simulink model "bldc_sim_combined_2024"  (R2025a)
settings: Solver=VariableStepAuto  StartTime=0.0  StopTime=1.5  RelTol=1e-3
values from neighbouring files (symbols this model uses):
  phi_corr_LUT_param = Simulink.Parameter(phi_corr_LUT)    [lut_script.m]
undefined symbols (not defined in the file or in its folder): closed_loop, D_duty_cycle, D_m, DiscIntNeverNeededParam, hall_errors, I_duty_cycle, J_t, L_ss, lambda_m, P, P_duty_cycle, r_s, R_vs, T_m, theta_v, use_LUT, V_bus
libraries: spsMosfetLib x6, spsSeriesRLCBranchLib x4, spsVoltageMeasurementLib x3, spsControlledCurrentSourceLib x3, slpidlib x2, eeGeneralControl x1, simulink x1, embmathops x1, spsControlledVoltageSourceLib x1, spsPWMGeneratorDCDCLib x1, spsDCVoltageSourceLib x1, sps_lib x1
(part 1 of 2)
settings Model: Creator=Aether  LastModifiedBy=rnashota.stu

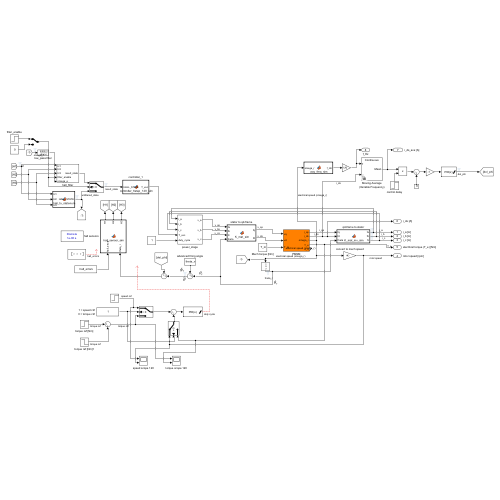
[thumbnail: Simulink's stored preview of the top-level diagram]
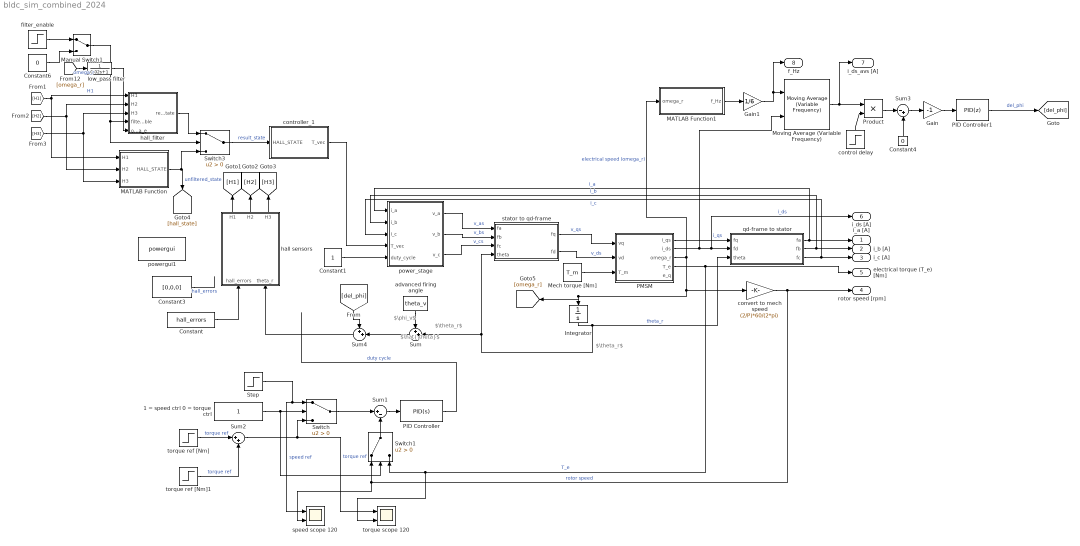
== system bldc_sim_combined_2024 ==
  note: $\theta_r$
  note: $\hat{\theta}$
  note: $\theta_r$
  note: $\phi_v$
  1 = speed ctrl 0 = torque ctrl : Constant
  Constant : Constant  Value=hall_errors
  Constant1 : Constant
  Constant3 : Constant  Value=[0,0,0]
  Constant4 : Constant  Value=0
  Constant6 : Constant  Value=0
  Gain : Gain  Gain=-1
  Gain1 : Gain  Gain=1/6
  Integrator : Integrator
  MATLAB Function : MATLAB Function  TreatAsAtomicUnit=on
  MATLAB Function1 : MATLAB Function  TreatAsAtomicUnit=on
  Manual Switch1 : ManualSwitch
  Mech torque [Nm] : Constant  Value=T_m
  Moving Average (Variable Frequency) : eeGeneralControl/Moving Average (Variable Frequency)  VariantControl=Variant1  LabelModeActiveChoice=Continuous  f0=60  fmin=1  x0=0  BufferSize=32768  Ts=0
      settings: LibrarySourceBlock=|
      | ee_sl_lib/General Control/Moving Average
      | (Variable Frequency)
  PID Controller : slpidlib/PID Controller  Controller=PID  Form=Parallel  TimeDomain=Continuous-time  UseExternalTs=off  SampleTime=-1  IntegratorMethod=Forward Euler  FilterMethod=Forward Euler  ControllerParametersSource=internal  P=P_duty_cycle  I=I_duty_cycle  UseKiTs=off  D=D_duty_cycle  UseExternalDerivativeSource=off  N=100  UseFilter=on  TunerSelectOption=Transfer Function Based (PID Tuner App)  InitialConditionSource=internal  InitialConditionForIntegrator=0  InitialConditionForFilter=0  DifferentiatorICPrevScaledInput=0  ExternalReset=none  TrackingMode=off  Kt=1  LimitOutput=on  SatLimitsSource=internal  UpperSaturationLimit=1  LowerSaturationLimit=0  LinearizeAsGain=on  AntiWindupMode=none  Kb=1  LimitIntegrator=off  UpperIntegratorSaturationLimit=inf  LowerIntegratorSaturationLimit=-inf  POutMin=[]  POutMax=[]  IOutMin=[]  IOutMax=[]  DOutMin=[]  DOutMax=[]  NOutMin=[]  NOutMax=[]  SumOutMin=[]  SumOutMax=[]  SaturationOutMin=[]  SaturationOutMax=[]  PParamMin=[]  PParamMax=[]  IParamMin=[]  IParamMax=[]  DParamMin=[]  DParamMax=[]  NParamMin=[]  NParamMax=[]  KbParamMin=[]  KbParamMax=[]  KtParamMin=[]  KtParamMax=[]  KbOutMin=[]  KbOutMax=[]  KtOutMin=[]  KtOutMax=[]  IntegratorOutMin=[]  IntegratorOutMax=[]  FilterOutMin=[]  FilterOutMax=[]  SumI1OutMin=[]  SumI1OutMax=[]  SumI2OutMin=[]  SumI2OutMax=[]  SumI3OutMin=[]  SumI3OutMax=[]  SumI4OutMin=[]  SumI4OutMax=[]  SumDOutMin=[]  SumDOutMax=[]  DifferentiatorOutMin=[]  DifferentiatorOutMax=[]  FilterDiffOutCoefMin=[]  FilterDiffOutCoefMax=[]  ReciprocalOutMin=[]  ReciprocalOutMax=[]  SumDenOutMin=[]  SumDenOutMax=[]  SumNumOutMin=[]  SumNumOutMax=[]  DivideOutMin=[]  DivideOutMax=[]  UdiffTsProdOutMin=[]  UdiffTsProdOutMax=[]  NTsProdOutMin=[]  NTsProdOutMax=[]  UintegralTsProdOutMin=[]  UintegralTsProdOutMax=[]  UngainTsProdOutMin=[]  UngainTsProdOutMax=[]  ClampingZeroOutDataTypeStr=Inherit: Inherit via back propagation  ClampingZeroOutMin=[]  ClampingZeroOutMax=[]  FilterDenConstantOutDataTypeStr=Inherit: Inherit via back propagation  FilterDenConstantOutMin=[]  FilterDenConstantOutMax=[]  PCopyOutDataTypeStr=Inherit: Inherit via back propagation  PCopyOutMin=[]  PCopyOutMax=[]  NCopyOutDataTypeStr=Inherit: Inherit via back propagation  NCopyOutMin=[]  NCopyOutMax=[]  IntegratorContinuousStateAttributes=''  IntegratorStateMustResolveToSignalObject=off  IntegratorRTWStateStorageClass=Auto  FilterContinuousStateAttributes=''  FilterStateMustResolveToSignalObject=off  FilterRTWStateStorageClass=Auto  ParallelPVariant=InternalParameters  IdealPVariant=Disabled  IVariant=InternalParameters  DVariant=InternalParameters  IntegratorVariant=Continuous  SatVariant=Enabled  AWVariant=Passthrough  PCopyVariant=Disabled  TRVariant=Disabled  FdbkBlocksVariant=Forward  IdealPFdbkVariant=Disabled  SatFdbkVariant=Disabled  DerivativeFilterVariant=ContFilter  NVariant=InternalParameters  NCopyVariant=Disabled  FilterICVariant=InternalICsFilter  IntegratorICVariant=InternalICs  ExternalResetVariant=Disabled  TRSumVariant=Passthrough  SumFdbkVariant=Disabled  SumVariant=Sum_PID  TsampFilterVariant=InternalTs  TsampNgainVariant=Passthrough  TsampIntegralVariant=Disabled_SignalSpec  ExternalSaturationOutDataTypeStr=Inherit: Same as second input  DerivativeSourceVariant=ErrorSignal  PreIntVariant=InternalPreInt
  PID Controller1 : slpidlib/PID Controller  Controller=PID  Form=Parallel  TimeDomain=Discrete-time  UseExternalTs=off  SampleTime=-1  IntegratorMethod=Forward Euler  FilterMethod=Forward Euler  ControllerParametersSource=internal  P=0.0068  I=0.744  UseKiTs=off  D=0  UseExternalDerivativeSource=off  N=100  UseFilter=on  TunerSelectOption=Transfer Function Based (PID Tuner App)  InitialConditionSource=internal  InitialConditionForIntegrator=0  InitialConditionForFilter=0  DifferentiatorICPrevScaledInput=0  ExternalReset=none  TrackingMode=off  Kt=1  LimitOutput=on  SatLimitsSource=internal  UpperSaturationLimit=pi/3  LowerSaturationLimit=-pi/3  LinearizeAsGain=on  AntiWindupMode=none  Kb=1  LimitIntegrator=off  UpperIntegratorSaturationLimit=inf  LowerIntegratorSaturationLimit=-inf  POutMin=[]  POutMax=[]  IOutMin=[]  IOutMax=[]  DOutMin=[]  DOutMax=[]  NOutMin=[]  NOutMax=[]  SumOutMin=[]  SumOutMax=[]  SaturationOutMin=[]  SaturationOutMax=[]  PParamMin=[]  PParamMax=[]  IParamMin=[]  IParamMax=[]  DParamMin=[]  DParamMax=[]  NParamMin=[]  NParamMax=[]  KbParamMin=[]  KbParamMax=[]  KtParamMin=[]  KtParamMax=[]  KbOutMin=[]  KbOutMax=[]  KtOutMin=[]  KtOutMax=[]  IntegratorOutMin=[]  IntegratorOutMax=[]  FilterOutMin=[]  FilterOutMax=[]  SumI1OutMin=[]  SumI1OutMax=[]  SumI2OutMin=[]  SumI2OutMax=[]  SumI3OutMin=[]  SumI3OutMax=[]  SumI4OutMin=[]  SumI4OutMax=[]  SumDOutMin=[]  SumDOutMax=[]  DifferentiatorOutMin=[]  DifferentiatorOutMax=[]  FilterDiffOutCoefMin=[]  FilterDiffOutCoefMax=[]  ReciprocalOutMin=[]  ReciprocalOutMax=[]  SumDenOutMin=[]  SumDenOutMax=[]  SumNumOutMin=[]  SumNumOutMax=[]  DivideOutMin=[]  DivideOutMax=[]  UdiffTsProdOutMin=[]  UdiffTsProdOutMax=[]  NTsProdOutMin=[]  NTsProdOutMax=[]  UintegralTsProdOutMin=[]  UintegralTsProdOutMax=[]  UngainTsProdOutMin=[]  UngainTsProdOutMax=[]  ClampingZeroOutDataTypeStr=Inherit: Inherit via back propagation  ClampingZeroOutMin=[]  ClampingZeroOutMax=[]  FilterDenConstantOutDataTypeStr=Inherit: Inherit via back propagation  FilterDenConstantOutMin=[]  FilterDenConstantOutMax=[]  PCopyOutDataTypeStr=Inherit: Inherit via back propagation  PCopyOutMin=[]  PCopyOutMax=[]  NCopyOutDataTypeStr=Inherit: Inherit via back propagation  NCopyOutMin=[]  NCopyOutMax=[]  IntegratorContinuousStateAttributes=''  IntegratorStateMustResolveToSignalObject=off  IntegratorRTWStateStorageClass=Auto  FilterContinuousStateAttributes=''  FilterStateMustResolveToSignalObject=off  FilterRTWStateStorageClass=Auto  ParallelPVariant=InternalParameters  IdealPVariant=Disabled  IVariant=InternalParameters  DVariant=InternalParameters  IntegratorVariant=Discrete  SatVariant=Enabled  AWVariant=Passthrough  PCopyVariant=Disabled  TRVariant=Disabled  FdbkBlocksVariant=Forward  IdealPFdbkVariant=Disabled  SatFdbkVariant=Disabled  DerivativeFilterVariant=ForwardEulerFilter  NVariant=InternalParameters  NCopyVariant=Disabled  FilterICVariant=InternalICsFilter  IntegratorICVariant=InternalICs  ExternalResetVariant=Disabled  TRSumVariant=Passthrough  SumFdbkVariant=Disabled  SumVariant=Sum_PID  TsampFilterVariant=InternalTs  TsampNgainVariant=Passthrough  TsampIntegralVariant=Disabled_SignalSpec  ExternalSaturationOutDataTypeStr=Inherit: Same as second input  DerivativeSourceVariant=ErrorSignal  PreIntVariant=InternalPreInt
  PMSM : Subsystem
  Product : Product
  Step : Step  Time=0.1  After=1000  SampleTime=0
  Sum : Sum  Inputs=++|
  Sum1 : Sum  Inputs=|+-
  Sum2 : Sum  Inputs=|++
  Sum3 : Sum  Inputs=|-+
  Sum4 : Sum  Inputs=++|
  Switch : Switch  Criteria=u2 > Threshold  SaturateOnIntegerOverflow=off  InputSameDT=off
  Switch1 : Switch  Criteria=u2 > Threshold  SaturateOnIntegerOverflow=off  InputSameDT=off
  Switch3 : Switch  Criteria=u2 > Threshold  SaturateOnIntegerOverflow=off  InputSameDT=off
  advanced firing angle : Constant  Value=theta_v
  control delay : Step  Time=0.6  SampleTime=0
  controller_1 : MATLAB Function  TreatAsAtomicUnit=on
  convert to mech speed : Gain  Gain=(2/P)*60/(2*pi)
  filter_enable : Step  Time=0.5  SampleTime=0
  hall sensors : MATLAB Function  TreatAsAtomicUnit=on
  hall_filter : Subsystem
  low_pass filter : TransferFcn  Denominator=[0.02 1]
  power_stage : Subsystem
  powergui1 : sps_lib/powergui  Priority=1  SimulationMode=Discrete  SampleTime=1e-6  frequency=60  Iterations=50  frequencyindice=0  Pbase=100e6  ErrMax=1e-4  UnitsV=kV  UnitsW=MW  buscounter=0  FunctionMessages=off  echomessages=off  EnableUseOfTLC=off  CurrentSourceSwitches=off  DisableSnubberDevices=off  DisableRonSwitches=off  DisableVfSwitches=off  DisplayEquations=off  AutomaticDiscreteSolvers=off  SolverType=Tustin/Backward Euler (TBE)  Interpol=off  ExternalGateDelay=off  methode=off  Ts=100  x0status=blocks  SPID=on  SwTol=0  HookPort=off  NonlinearTolerance=1e-4  nMaxIteration=100  ContinueOnMaxIteration=off  RestoreLinks=warning  ResistiveCurrentMeasurement=off  Frange=[0:2:500]  Ylog=off  Xlog=on  ShowGrid=off  save=off  variable=ZData  structure=0  ZoomFFT=off  StartTime=0.0  cycles=1  DisplayStyle=1  fundamental=60  FreqAxis=off  MaxFrequency=1000  frequencyindicesteady=1  RmsSteady=1  display=off
  qd-frame to stator : MATLAB Function  TreatAsAtomicUnit=on
  speed scope 120 : Scope  NumInputPorts=2
      settings: ActiveDisplayYMinimum=-1.1385486491945782E+15  ActiveDisplayYMaximum=1.0246937842751196E+16
  stator to qd-frame : MATLAB Function  TreatAsAtomicUnit=on
  torque ref [Nm] : Step  Time=0.1  After=1e-1  SampleTime=0  ZeroCross=off
  torque ref [Nm]1 : Step  After=-0.5e-1  SampleTime=0
  torque scope 120 : Scope  NumInputPorts=2
      settings: ActiveDisplayYMinimum=-0.89883  ActiveDisplayYMaximum=8.08945
  i_a [A] : Outport
  i_b [A] : Outport  Port=2
  i_c [A] : Outport  Port=3
  rotor speed [rpm] : Outport  Port=4
  electrical torque (T_e) [Nm] : Outport  Port=5
  i_ds [A] : Outport  Port=6
  i_ds_avs [A] : Outport  Port=7
  f_Hz : Outport  Port=8
  wires:
  Constant3/1 -> ?  "hall_errors"
  qd-frame to stator/2(fb) -> power_stage/2(i_b), i_b [A]/1  "i_b"
  qd-frame to stator/3(fc) -> power_stage/3(i_c), i_c [A]/1  "i_c"
  power_stage/1(v_a) -> stator to qd-frame/1(fa)  "v_as"
  Sum/1 -> Sum4/2
  PMSM/3(omega_r) -> MATLAB Function1/1(omega_r), convert to mech speed/1, [omega_r], Integrator/1  "electrical speed (omega_r)"
  Sum4/1 -> hall sensors/2(theta_r)
  advanced firing angle/1 -> Sum/1
  qd-frame to stator/1(fa) -> power_stage/1(i_a), i_a [A]/1  "i_a"
  Integrator/1 -> stator to qd-frame/4(theta), Sum/2, qd-frame to stator/3(theta)  "theta_r"
  power_stage/2(v_b) -> stator to qd-frame/2(fb)  "v_bs"
  stator to qd-frame/2(fd) -> PMSM/2(vd)  "v_ds"
  power_stage/3(v_c) -> stator to qd-frame/3(fc)  "v_cs"
  Mech torque [Nm]/1 -> PMSM/3(T_m)
  stator to qd-frame/1(fq) -> PMSM/1(vq)  "v_qs"
  PMSM/1(i_qs) -> qd-frame to stator/1(fq)  "i_qs"
  Product/1 -> Sum3/1
  Gain/1 -> PID Controller1/1
  Sum3/1 -> Gain/1
  PID Controller1/1 -> [del_phi]  "del_phi"
  Moving Average (Variable Frequency)/1 -> Product/1, i_ds_avs [A]/1
  PMSM/2(i_ds) -> qd-frame to stator/2(fd), i_ds [A]/1, Moving Average (Variable Frequency)/2  "i_ds"
  Constant4/1 -> Sum3/2
  control delay/1 -> Product/2
  [del_phi] -> Sum4/1
  Step/1 -> speed scope 120/1, Switch/1  "speed ref"
  1 = speed ctrl 0 = torque ctrl/1 -> Switch/2, Switch1/2
  Switch/1 -> Sum1/1
  Switch1/1 -> Sum1/2
  torque ref [Nm]/1 -> Sum2/1  "torque ref"
  PMSM/4(T_e) -> torque scope 120/2, Switch1/3, electrical torque (T_e) [Nm]/1  "T_e"
  Sum1/1 -> PID Controller/1
  torque ref [Nm]1/1 -> Sum2/2  "torque ref"
  convert to mech speed/1 -> rotor speed [rpm]/1, Switch1/1, speed scope 120/2  "rotor speed"
  Sum2/1 -> torque scope 120/1, Switch/3  "torque ref"
  MATLAB Function1/1(f_Hz) -> Gain1/1
  Gain1/1 -> Moving Average (Variable Frequency)/1, f_Hz/1
  Constant1/1 -> power_stage/5(duty_cycle)
  Constant/1 -> hall sensors/1(hall_errors)
  hall sensors/1(H1) -> [H1]
  hall sensors/2(H2) -> [H2]
  hall sensors/3(H3) -> [H3]
  filter_enable/1 -> Manual Switch1/1
  Constant6/1 -> Manual Switch1/2
  MATLAB Function/1(HALL_STATE) -> [hall_state], Switch3/3  "unfiltered_state"
  [H3] -> hall_filter/3(H3), MATLAB Function/3(H3)
  hall_filter/1(result_state) -> Switch3/1
  [H2] -> hall_filter/2(H2), MATLAB Function/2(H2)
  Manual Switch1/1 -> Switch3/2, hall_filter/4(filter_enable)
  [H1] -> hall_filter/1(H1), MATLAB Function/1(H1)  "H1"
  Switch3/1 -> controller_1/1(HALL_STATE)  "result_state"
  controller_1/1(T_vec) -> power_stage/4(T_vec)
  PID Controller/1 -> ?  "duty cycle"
  [omega_r] -> low_pass filter/1  "omega_r"
  low_pass filter/1 -> hall_filter/5(omega_e)

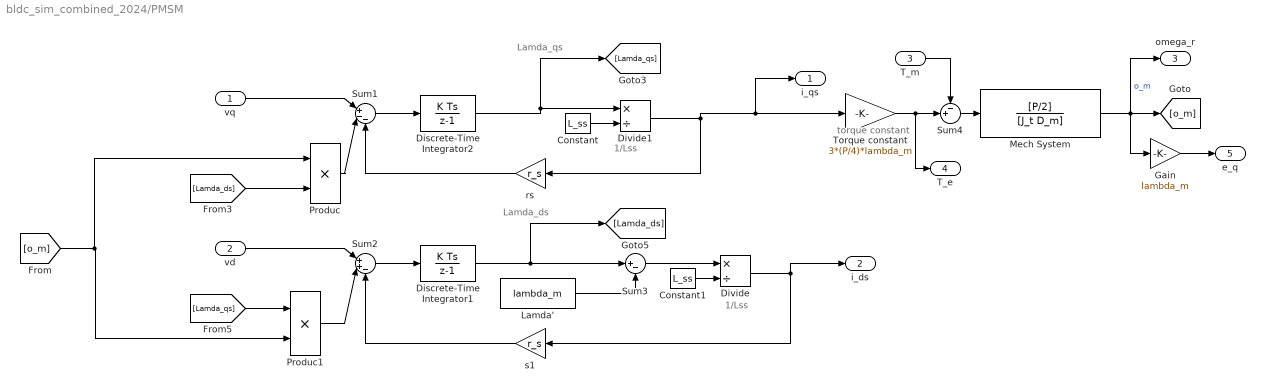
== system bldc_sim_combined_2024/PMSM ==
  note: torque constant
  note: Lamda_ds
  note: Lamda_qs
  note: 1/Lss
  note: 1/Lss
  vq : Inport
  vd : Inport  Port=2
  T_m : Inport  Port=3
  Constant : Constant  Value=L_ss
  Constant1 : Constant  Value=L_ss
  Discrete-Time Integrator1 : DiscreteIntegrator  SampleTime=-1  ICPrevOutput=DiscIntNeverNeededParam  ICPrevScaledInput=DiscIntNeverNeededParam
  Discrete-Time Integrator2 : DiscreteIntegrator  SampleTime=-1  ICPrevOutput=DiscIntNeverNeededParam  ICPrevScaledInput=DiscIntNeverNeededParam
  Divide : Product  Inputs=*/
  Divide1 : Product  Inputs=*/
  Gain : Gain  Gain=lambda_m
  Lamda' : Constant  Value=lambda_m
  Mech System : TransferFcn  Numerator=[P/2]  Denominator=[J_t D_m]
  Produc : Product  RndMeth=Zero
  Produc1 : Product  RndMeth=Zero
  Sum1 : Sum  Inputs=|+--
  Sum2 : Sum  Inputs=|++-
  Sum3 : Sum  Inputs=|+-
  Sum4 : Sum  Inputs=-+|
  Torque constant : Gain  Gain=3*(P/4)*lambda_m
  rs : Gain  Gain=r_s
  s1 : Gain  Gain=r_s
  i_qs : Outport
  i_ds : Outport  Port=2
  omega_r : Outport  Port=3
  T_e : Outport  Port=4
  e_q : Outport  Port=5
  wires:
  vd/1 -> Sum2/1
  vq/1 -> Sum1/1
  [Lamda_qs] -> Produc1/1
  [Lamda_ds] -> Produc/2
  [o_m] -> Produc1/2, Produc/1
  Lamda'/1 -> Sum3/2
  Sum3/1 -> Divide/1
  s1/1 -> Sum2/3
  Discrete-Time Integrator1/1 -> [Lamda_ds], Sum3/1
  Sum2/1 -> Discrete-Time Integrator1/1
  Produc1/1 -> Sum2/2
  Divide1/1 -> i_qs/1, Torque constant/1, rs/1
  rs/1 -> Sum1/3
  Discrete-Time Integrator2/1 -> [Lamda_qs], Divide1/1
  Sum1/1 -> Discrete-Time Integrator2/1
  Produc/1 -> Sum1/2
  Torque constant/1 -> Sum4/2, T_e/1
  Divide/1 -> i_ds/1, s1/1
  T_m/1 -> Sum4/1
  Sum4/1 -> Mech System/1
  Constant/1 -> Divide1/2
  Constant1/1 -> Divide/2
  Mech System/1 -> Gain/1, omega_r/1, [o_m]  "o_m"
  Gain/1 -> e_q/1

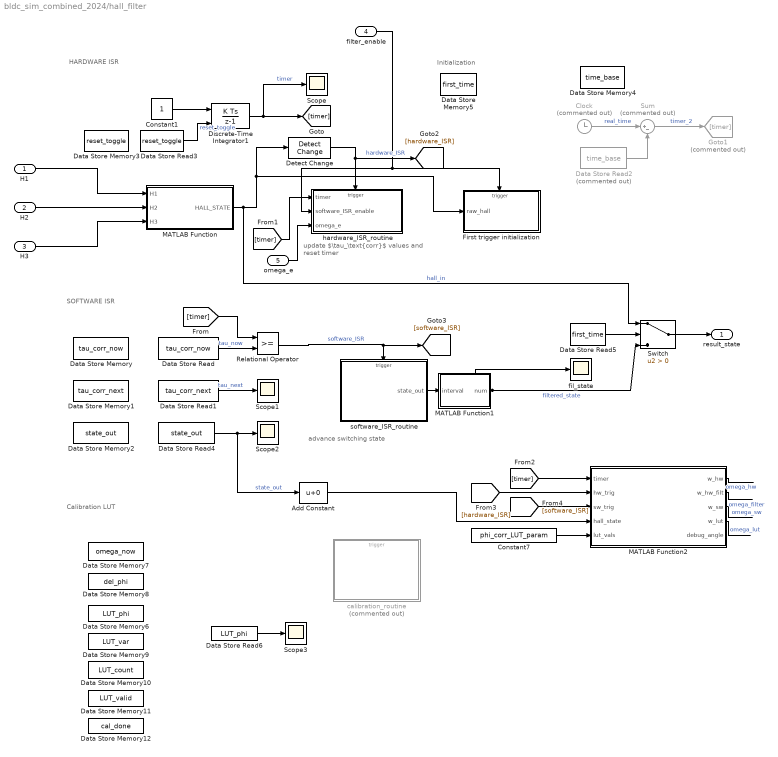
== system bldc_sim_combined_2024/hall_filter ==
  note: Calibration LUT
  note: Initialization
  note: SOFTWARE ISR
  note: HARDWARE ISR
  note: update $\tau_\text{corr}$ values and reset timer
  note: advance switching state
  H1 : Inport
  H2 : Inport  Port=2
  H3 : Inport  Port=3
  filter_enable : Inport  Port=4
  omega_e : Inport  Port=5
  Add Constant : Bias  SaturateOnIntegerOverflow=off
  Clock : Clock  Commented=on
  Constant1 : Constant
  Constant7 : Constant  Value=phi_corr_LUT_param
  Data Store Memory : DataStoreMemory  DataStoreName=tau_corr_now  WriteAfterWriteMsg=warning  InitialValue=-1  ShowAdditionalParam=off
  Data Store Memory1 : DataStoreMemory  DataStoreName=tau_corr_next  WriteAfterWriteMsg=warning  InitialValue=-1  ShowAdditionalParam=off
  Data Store Memory10 : DataStoreMemory  DataStoreName=LUT_count  WriteAfterWriteMsg=warning  InitialValue=[0 0 0 0 0 0]  ShowAdditionalParam=off
  Data Store Memory11 : DataStoreMemory  DataStoreName=LUT_valid  WriteAfterWriteMsg=warning  InitialValue=[0 0 0 0 0 0]  ShowAdditionalParam=off
  Data Store Memory12 : DataStoreMemory  DataStoreName=cal_done  WriteAfterWriteMsg=warning  ShowAdditionalParam=off  OutDataTypeStr=boolean
  Data Store Memory2 : DataStoreMemory  DataStoreName=state_out  WriteAfterWriteMsg=warning  InitialValue=2  ShowAdditionalParam=off
  Data Store Memory3 : DataStoreMemory  DataStoreName=reset_toggle  WriteAfterWriteMsg=warning  ShowAdditionalParam=off
  Data Store Memory4 : DataStoreMemory  DataStoreName=time_base  WriteAfterWriteMsg=warning  ShowAdditionalParam=off
  Data Store Memory5 : DataStoreMemory  DataStoreName=first_time  WriteAfterWriteMsg=warning  InitialValue=1  ShowAdditionalParam=off
  Data Store Memory6 : DataStoreMemory  DataStoreName=LUT_phi  WriteAfterWriteMsg=warning  InitialValue=[0 0 0 0 0 0]  ShowAdditionalParam=off
  Data Store Memory7 : DataStoreMemory  DataStoreName=omega_now  WriteAfterWriteMsg=warning  ShowAdditionalParam=off
  Data Store Memory8 : DataStoreMemory  DataStoreName=del_phi  WriteAfterWriteMsg=warning  ShowAdditionalParam=off
  Data Store Memory9 : DataStoreMemory  DataStoreName=LUT_var  WriteAfterWriteMsg=warning  InitialValue=[0 0 0 0 0 0]  ShowAdditionalParam=off
  Data Store Read : DataStoreRead  DataStoreName=tau_corr_now  IndexOptions=Index vector (dialog)  Indices=1  OutputSizes=1
  Data Store Read1 : DataStoreRead  DataStoreName=tau_corr_next  IndexOptions=Index vector (dialog)  Indices=1  OutputSizes=1
  Data Store Read2 : DataStoreRead  Commented=on  DataStoreName=time_base  IndexOptions=Index vector (dialog)  Indices=1  OutputSizes=1
  Data Store Read3 : DataStoreRead  DataStoreName=reset_toggle  IndexOptions=Index vector (dialog)  Indices=1  OutputSizes=1
  Data Store Read4 : DataStoreRead  DataStoreName=state_out  IndexOptions=Index vector (dialog)  Indices=1  OutputSizes=1
  Data Store Read5 : DataStoreRead  DataStoreName=first_time  IndexOptions=Index vector (dialog)  Indices=1  OutputSizes=1
  Data Store Read6 : DataStoreRead  DataStoreName=LUT_phi  IndexOptions=Index vector (dialog)  Indices=1  OutputSizes=1
  Detect Change : simulink/Logic and Bit Operations/Detect Change  vinit=0  OutDataTypeStr=boolean
  Discrete-Time Integrator1 : DiscreteIntegrator  ExternalReset=either  SampleTime=1/(1e6)  ICPrevOutput=DiscIntNeverNeededParam  ICPrevScaledInput=DiscIntNeverNeededParam
  First trigger initialization : Subsystem  TreatAsAtomicUnit=on
  Goto1 : Goto  Commented=on  GotoTag=timer
  MATLAB Function : MATLAB Function  TreatAsAtomicUnit=on
  MATLAB Function1 : MATLAB Function  TreatAsAtomicUnit=on
  MATLAB Function2 : MATLAB Function  TreatAsAtomicUnit=on  SystemSampleTime=1e-6
  Relational Operator : RelationalOperator  OutDataTypeStr=boolean  RndMeth=Simplest  InputSameDT=off
  Scope{,1..3} (4 alike) : Scope
      Scope settings: ActiveDisplayYMinimum=-6.25  ActiveDisplayYMaximum=56.25
      Scope1 settings: ActiveDisplayYMinimum=7.96701  ActiveDisplayYMaximum=8.03137
      Scope2 settings: ActiveDisplayYMinimum=7.96701  ActiveDisplayYMaximum=8.03137
      Scope3 settings: ActiveDisplayYMinimum=0.99241576103971962  ActiveDisplayYMaximum=1.0799572702760518  DataLoggingVariableName=ScopeData2
  Sum : Sum  Commented=on  Inputs=|+-
  Switch : Switch  Criteria=u2 > Threshold  SaturateOnIntegerOverflow=off  InputSameDT=off
  calibration_routine : Subsystem  Priority=11  Commented=on  TreatAsAtomicUnit=on
  fil_state : Scope
      settings: ActiveDisplayYMinimum=-0.75  ActiveDisplayYMaximum=6.75  DataLoggingVariableName=ScopeData3
  hardware_ISR_routine : Subsystem  Priority=1
  software_ISR_routine : Subsystem  Priority=10  TreatAsAtomicUnit=on
  result_state : Outport
  wires:
  Discrete-Time Integrator1/1 -> [timer], Scope/1  "timer"
  Relational Operator/1 -> [software_ISR], software_ISR_routine/Trigger  "software_ISR"
  Constant1/1 -> Discrete-Time Integrator1/1
  [timer] -> Relational Operator/1
  software_ISR_routine/1(state_out) -> MATLAB Function1/1(interval)
  MATLAB Function/1(HALL_STATE) -> Switch/1, Detect Change/1, First trigger initialization/1(raw_hall)  "hall_in"
  Data Store Read3/1 -> Discrete-Time Integrator1/2  "reset_toggle"
  Data Store Read1/1 -> Scope1/1  "tau_next"
  Data Store Read/1 -> Relational Operator/2  "tau_now"
  H3/1 -> MATLAB Function/3(H3)
  H2/1 -> MATLAB Function/2(H2)
  H1/1 -> MATLAB Function/1(H1)
  MATLAB Function1/1(num) -> fil_state/1, Switch/3  "filtered_state"
  Detect Change/1 -> [hardware_ISR], hardware_ISR_routine/Trigger  "hardware_ISR"
  Data Store Read4/1 -> Add Constant/1, Scope2/1  "state_out"
  filter_enable/1 -> First trigger initialization/Trigger, hardware_ISR_routine/2(software_ISR_enable)
  Clock/1 -> Sum/1  "real_time"
  [timer] -> hardware_ISR_routine/1(timer)
  Data Store Read2/1 -> Sum/2
  Sum/1 -> Goto1/1  "timer_2"
  Data Store Read5/1 -> Switch/2
  Switch/1 -> result_state/1
  Data Store Read6/1 -> Scope3/1
  omega_e/1 -> hardware_ISR_routine/3(omega_e)
  [timer] -> MATLAB Function2/1(timer)
  [hardware_ISR] -> MATLAB Function2/2(hw_trig)
  [software_ISR] -> MATLAB Function2/3(sw_trig)
  Add Constant/1 -> MATLAB Function2/4(hall_state)
  Constant7/1 -> MATLAB Function2/5(lut_vals)
  MATLAB Function2/1(w_hw) -> ?  "omega_hw"
  MATLAB Function2/2(w_hw_filt) -> ?  "omega_filter"
  MATLAB Function2/3(w_sw) -> ?  "omega_sw"
  MATLAB Function2/4(w_lut) -> ?  "omega_lut"

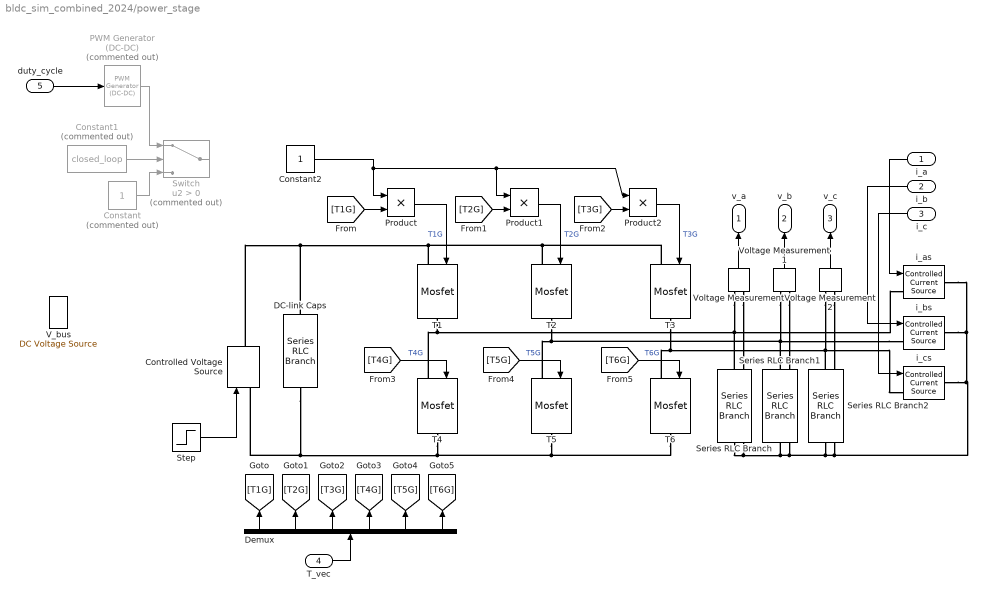
== system bldc_sim_combined_2024/power_stage ==
  i_a : Inport
  i_b : Inport  Port=2
  i_c : Inport  Port=3
  T_vec : Inport  Port=4
  duty_cycle : Inport  Port=5
  Constant : Constant  Commented=on
  Constant1 : Constant  Commented=on  Value=closed_loop
  Constant2 : Constant
  Controlled Voltage Source : spsControlledVoltageSourceLib/Controlled Voltage Source  Initialize=on  Source_Type=DC  Amplitude=20  Phase=0  Frequency=0  Measurements=None
  DC-link Caps : spsSeriesRLCBranchLib/Series RLC Branch  LConnTagsString=__new0  RConnTagsString=__new0  BranchType=RC  Resistance=1e-6  Inductance=0  SetiL0=off  InitialCurrent=0  Capacitance=100e-6  Setx0=off  InitialVoltage=0  Measurements=None
  Demux : Demux  Outputs=6
  PWM Generator (DC-DC) : spsPWMGeneratorDCDCLib/PWM Generator (DC-DC)  Commented=on  Fsw=f_SW_Hz  Ts=0
  Product : Product
  Product1 : Product
  Product2 : Product
  Series RLC Branch : spsSeriesRLCBranchLib/Series RLC Branch  LConnTagsString=__new0  RConnTagsString=__new0  BranchType=R  Resistance=R_vs  Inductance=0  SetiL0=off  InitialCurrent=0  Capacitance=inf  Setx0=off  InitialVoltage=0  Measurements=None
  Series RLC Branch1 : spsSeriesRLCBranchLib/Series RLC Branch  LConnTagsString=__new0  RConnTagsString=__new0  BranchType=R  Resistance=R_vs  Inductance=0  SetiL0=off  InitialCurrent=0  Capacitance=inf  Setx0=off  InitialVoltage=0  Measurements=None
  Series RLC Branch2 : spsSeriesRLCBranchLib/Series RLC Branch  LConnTagsString=__new0  RConnTagsString=__new0  BranchType=R  Resistance=R_vs  Inductance=0  SetiL0=off  InitialCurrent=0  Capacitance=inf  Setx0=off  InitialVoltage=0  Measurements=None
  Step : Step  Time=0.55  Before=20  After=35  SampleTime=0
  Switch : Switch  Commented=on  Criteria=u2 > Threshold  SaturateOnIntegerOverflow=off  InputSameDT=off
  T{1..6} (6 alike) : spsMosfetLib/Mosfet  Ron=R_dsON_Ohm  Lon=0  Rd=0.01  Vfd=0.7  IC=0  Rs=1e5  Cs=inf  Measurements=off
  V_bus : spsDCVoltageSourceLib/DC Voltage Source  Amplitude=V_bus  Measurements=None
  Voltage Measurement : spsVoltageMeasurementLib/Voltage Measurement  PhasorSimulation=off  OutputType=Complex  PSBequivalent=0
  Voltage Measurement1 : spsVoltageMeasurementLib/Voltage Measurement  PhasorSimulation=off  OutputType=Complex  PSBequivalent=0
  Voltage Measurement2 : spsVoltageMeasurementLib/Voltage Measurement  PhasorSimulation=off  OutputType=Complex  PSBequivalent=0
  i_as : spsControlledCurrentSourceLib/Controlled Current Source  Initialize=on  Source_Type=AC  Amplitude=0  Phase=0  Frequency=0  Measurements=None
  i_bs : spsControlledCurrentSourceLib/Controlled Current Source  Initialize=on  Source_Type=AC  Amplitude=0  Phase=0  Frequency=0  Measurements=None
  i_cs : spsControlledCurrentSourceLib/Controlled Current Source  Initialize=on  Source_Type=AC  Amplitude=0  Phase=0  Frequency=0  Measurements=None
  v_a : Outport
  v_b : Outport  Port=2
  v_c : Outport  Port=3
  wires:
  T_vec/1 -> Demux/1
  Product1/1 -> T2/1  "T2G"
  Constant2/1 -> Product/1, Product2/1, Product1/1
  Demux/6 -> [T6G]
  [T4G] -> T4/1  "T4G"
  [T5G] -> T5/1  "T5G"
  Demux/4 -> [T4G]
  Voltage Measurement/1 -> v_a/1
  [T2G] -> Product1/2
  Voltage Measurement1/1 -> v_b/1
  Voltage Measurement2/1 -> v_c/1
  i_a/1 -> i_as/1
  Demux/1 -> [T1G]
  Demux/5 -> [T5G]
  [T6G] -> T6/1  "T6G"
  i_c/1 -> i_cs/1
  Product/1 -> T1/1  "T1G"
  [T3G] -> Product2/2
  i_b/1 -> i_bs/1
  Product2/1 -> T3/1  "T3G"
  Demux/2 -> [T2G]
  Demux/3 -> [T3G]
  [T1G] -> Product/2
  duty_cycle/1 -> PWM Generator (DC-DC)/1
  Constant/1 -> Switch/3
  Constant1/1 -> Switch/2
  PWM Generator (DC-DC)/1 -> Switch/1
  Step/1 -> Controlled Voltage Source/1
  connections:
  i_bs/LConn1 -- Voltage Measurement1/LConn1 -- Series RLC Branch1/LConn1 -- T2/RConn1 -- T5/LConn1
  DC-link Caps/RConn1 -- Controlled Voltage Source/LConn1 -- T4/RConn1 -- T6/RConn1 -- T5/RConn1
  DC-link Caps/LConn1 -- Controlled Voltage Source/RConn1 -- T1/LConn1 -- T3/LConn1 -- T2/LConn1
  T4/LConn1 -- T1/RConn1 -- Voltage Measurement/LConn1 -- Series RLC Branch/LConn1 -- i_as/LConn1
  T3/RConn1 -- T6/LConn1 -- Voltage Measurement2/LConn1 -- Series RLC Branch2/LConn1 -- i_cs/LConn1
  Series RLC Branch/RConn1 -- Voltage Measurement/LConn2 -- i_bs/RConn1 -- i_as/RConn1 -- i_cs/RConn1 -- Voltage Measurement2/LConn2 -- Series RLC Branch2/RConn1 -- Voltage Measurement1/LConn2 -- Series RLC Branch1/RConn1

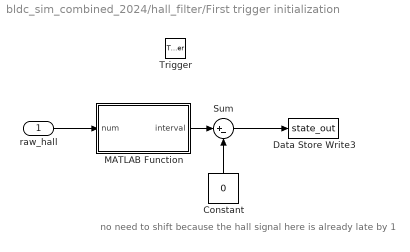
== system bldc_sim_combined_2024/hall_filter/First trigger initialization ==
  note: no need to shift because the hall signal here is already late by 1
  raw_hall : Inport
  Trigger : TriggerPort  VariantControl=(inherit)  PortDimensions=1
  Constant : Constant  Value=0
  Data Store Write3 : DataStoreWrite  DataStoreName=state_out  IndexOptions=Index vector (dialog)  Indices=1  OutputSizes=1
  MATLAB Function : MATLAB Function  TreatAsAtomicUnit=on
  Sum : Sum  Inputs=|+-
  wires:
  raw_hall/1 -> MATLAB Function/1(num)
  MATLAB Function/1(interval) -> Sum/1
  Sum/1 -> Data Store Write3/1
  Constant/1 -> Sum/2

== system bldc_sim_combined_2024/hall_filter/calibration_routine ==
  note: $calculate ~\omega$
  note: $calculate ~\Delta\phi$
  note: $update ~LUT ~ table$
  function : TriggerPort  VariantControl=(inherit)
  Subsystem : Subsystem  Priority=11
  Subsystem1 : Subsystem  Priority=12
  Subsystem2 : Subsystem  Priority=13

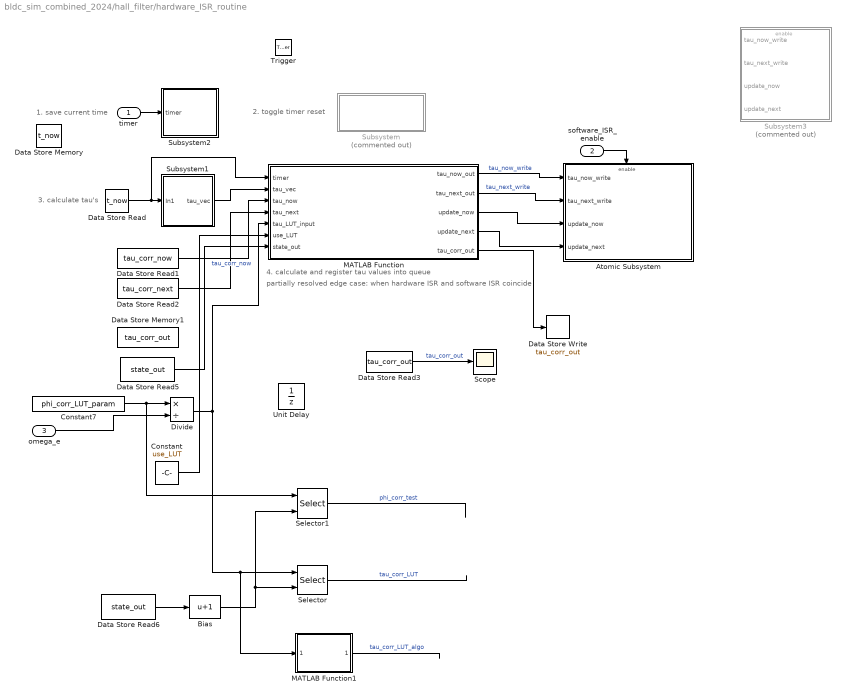
== system bldc_sim_combined_2024/hall_filter/hardware_ISR_routine ==
  note: partially resolved edge case: when hardware ISR and software ISR coincide
  note: 2. toggle timer reset
  note: 3. calculate tau's
  note: 4. calculate and register tau values into queue
  note: 1. save current time
  timer : Inport
  software_ISR_enable : Inport  Port=2
  omega_e : Inport  Port=3
  Trigger : TriggerPort  VariantControl=(inherit)  PortDimensions=1
  Atomic Subsystem : Subsystem  Priority=5  TreatAsAtomicUnit=on
  Bias : Bias  Bias=1  SaturateOnIntegerOverflow=off
  Constant : Constant  Value=use_LUT
  Constant7 : Constant  Value=phi_corr_LUT_param
  Data Store Memory : DataStoreMemory  DataStoreName=t_now  WriteAfterWriteMsg=warning  ShowAdditionalParam=off
  Data Store Memory1 : DataStoreMemory  DataStoreName=tau_corr_out  WriteAfterWriteMsg=warning  ShowAdditionalParam=off
  Data Store Read : DataStoreRead  DataStoreName=t_now  IndexOptions=Index vector (dialog)  Indices=1  OutputSizes=1
  Data Store Read1 : DataStoreRead  DataStoreName=tau_corr_now  IndexOptions=Index vector (dialog)  Indices=1  OutputSizes=1
  Data Store Read2 : DataStoreRead  DataStoreName=tau_corr_next  IndexOptions=Index vector (dialog)  Indices=1  OutputSizes=1
  Data Store Read3 : DataStoreRead  DataStoreName=tau_corr_out  IndexOptions=Index vector (dialog)  Indices=1  OutputSizes=1
  Data Store Read5 : DataStoreRead  DataStoreName=state_out  IndexOptions=Index vector (dialog)  Indices=1  OutputSizes=1
  Data Store Read6 : DataStoreRead  DataStoreName=state_out  IndexOptions=Index vector (dialog)  Indices=1  OutputSizes=1
  Data Store Write : DataStoreWrite  DataStoreName=tau_corr_out  IndexOptions=Index vector (dialog)  Indices=1  OutputSizes=1
  Divide : Product  Inputs=*/
  MATLAB Function : MATLAB Function  Priority=4  TreatAsAtomicUnit=on
  MATLAB Function1 : MATLAB Function  TreatAsAtomicUnit=on
  Scope : Scope
      settings: ActiveDisplayYMinimum=-0.027793962383284257  ActiveDisplayYMaximum=0.030008936086375265  DataLoggingVariableName=ScopeData4
  Selector : Selector  InputPortWidth=6  IndexOptions=Index vector (port)  Indices=[1 3]  OutputSizes=1
  Selector1 : Selector  InputPortWidth=6  IndexOptions=Index vector (port)  Indices=[1 3]  OutputSizes=1
  Subsystem : Subsystem  Priority=2  Commented=on
  Subsystem1 : Subsystem  Priority=3
  Subsystem2 : Subsystem  Priority=1
  Subsystem3 : Subsystem  Priority=5  Commented=on
  Unit Delay : UnitDelay  SampleTime=-1  HasFrameUpgradeWarning=on
  wires:
  Data Store Read/1 -> MATLAB Function/1(timer), Subsystem1/1(In1)
  Data Store Read1/1 -> MATLAB Function/3(tau_now)  "tau_corr_now"
  timer/1 -> Subsystem2/1(timer)
  Subsystem1/1(tau_vec) -> MATLAB Function/2(tau_vec)
  MATLAB Function/1(tau_now_out) -> Atomic Subsystem/1(tau_now_write)  "tau_now_write"
  MATLAB Function/2(tau_next_out) -> Atomic Subsystem/2(tau_next_write)  "tau_next_write"
  software_ISR_enable/1 -> Atomic Subsystem/Enable
  MATLAB Function/3(update_now) -> Atomic Subsystem/3(update_now)
  MATLAB Function/4(update_next) -> Atomic Subsystem/4(update_next)
  MATLAB Function/5(tau_corr_out) -> Data Store Write/1
  Data Store Read3/1 -> Scope/1  "tau_corr_out"
  Data Store Read2/1 -> MATLAB Function/4(tau_next)
  Constant/1 -> MATLAB Function/6(use_LUT)
  Constant7/1 -> Selector1/1, Divide/1
  Divide/1 -> MATLAB Function1/1(tau_LUT_input), Selector/1, MATLAB Function/5(tau_LUT_input)
  omega_e/1 -> Divide/2
  Bias/1 -> Selector1/2, Selector/2
  Selector/1 -> ?  "tau_corr_LUT"
  Data Store Read5/1 -> MATLAB Function/7(state_out)
  Selector1/1 -> ?  "phi_corr_test"
  Data Store Read6/1 -> Bias/1
  MATLAB Function1/1(tau_corr_LUT_test) -> ?  "tau_corr_LUT_algo"

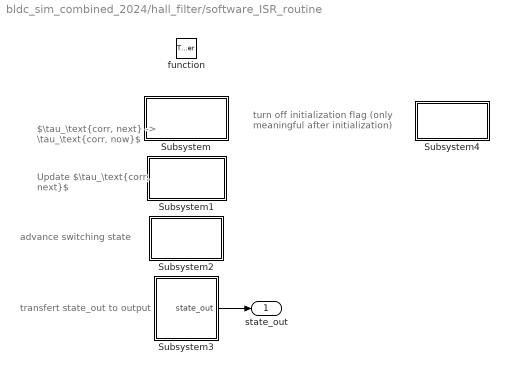
== system bldc_sim_combined_2024/hall_filter/software_ISR_routine ==
  note: turn off initialization flag
      | (only meaningful after initialization)
  note: advance switching state
  note: $\tau_\text{corr, next} -> \tau_\text{corr, now}$
  note: Update $\tau_\text{corr, next}$
  note: transfert state_out to output
  function : TriggerPort  VariantControl=(inherit)
  Subsystem : Subsystem  Priority=11
  Subsystem1 : Subsystem  Priority=12
  Subsystem2 : Subsystem  Priority=13
  Subsystem3 : Subsystem  Priority=14
  Subsystem4 : Subsystem  Priority=11
  state_out : Outport
  wires:
  Subsystem3/1(state_out) -> state_out/1

== system bldc_sim_combined_2024/hall_filter/calibration_routine/Subsystem ==
  Constant : Constant  Value=pi/3
  Data Store Read : DataStoreRead  DataStoreName=tau_corr_now  IndexOptions=Index vector (dialog)  Indices=1  OutputSizes=1
  Data Store Write : DataStoreWrite  DataStoreName=omega_now  IndexOptions=Index vector (dialog)  Indices=1  OutputSizes=1
  Divide : Product  Inputs=*/
  wires:
  Data Store Read/1 -> Divide/2
  Constant/1 -> Divide/1
  Divide/1 -> Data Store Write/1

== system bldc_sim_combined_2024/hall_filter/calibration_routine/Subsystem1 ==
  Data Store Read : DataStoreRead  DataStoreName=tau_corr_now  IndexOptions=Index vector (dialog)  Indices=1  OutputSizes=1
  Data Store Read1 : DataStoreRead  DataStoreName=omega_now  IndexOptions=Index vector (dialog)  Indices=1  OutputSizes=1
  Data Store Write : DataStoreWrite  DataStoreName=del_phi  IndexOptions=Index vector (dialog)  Indices=1  OutputSizes=1
  Product : Product
  wires:
  Data Store Read/1 -> Product/1
  Data Store Read1/1 -> Product/2
  Product/1 -> Data Store Write/1

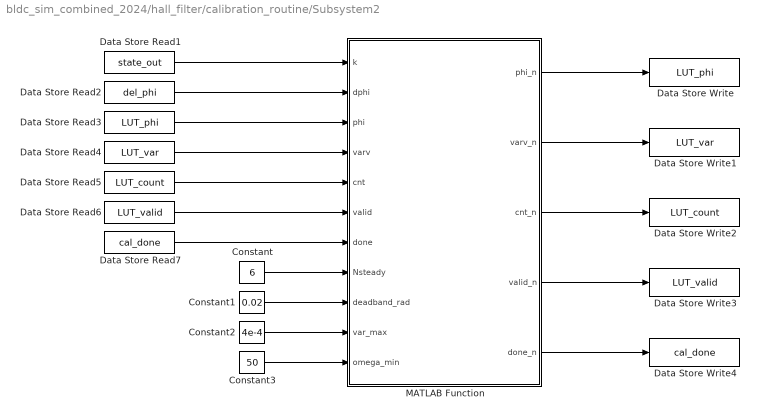
== system bldc_sim_combined_2024/hall_filter/calibration_routine/Subsystem2 ==
  Constant : Constant  Value=6
  Constant1 : Constant  Value=0.02
  Constant2 : Constant  Value=4e-4
  Constant3 : Constant  Value=50
  Data Store Read1 : DataStoreRead  DataStoreName=state_out  IndexOptions=Index vector (dialog)  Indices=1  OutputSizes=1
  Data Store Read2 : DataStoreRead  DataStoreName=del_phi  IndexOptions=Index vector (dialog)  Indices=1  OutputSizes=1
  Data Store Read3 : DataStoreRead  DataStoreName=LUT_phi  IndexOptions=Index vector (dialog)  Indices=1  OutputSizes=1
  Data Store Read4 : DataStoreRead  DataStoreName=LUT_var  IndexOptions=Index vector (dialog)  Indices=1  OutputSizes=1
  Data Store Read5 : DataStoreRead  DataStoreName=LUT_count  IndexOptions=Index vector (dialog)  Indices=1  OutputSizes=1
  Data Store Read6 : DataStoreRead  DataStoreName=LUT_valid  IndexOptions=Index vector (dialog)  Indices=1  OutputSizes=1
  Data Store Read7 : DataStoreRead  DataStoreName=cal_done  IndexOptions=Index vector (dialog)  Indices=1  OutputSizes=1
  Data Store Write : DataStoreWrite  DataStoreName=LUT_phi  IndexOptions=Index vector (dialog)  Indices=1  OutputSizes=1
  Data Store Write1 : DataStoreWrite  DataStoreName=LUT_var  IndexOptions=Index vector (dialog)  Indices=1  OutputSizes=1
  Data Store Write2 : DataStoreWrite  DataStoreName=LUT_count  IndexOptions=Index vector (dialog)  Indices=1  OutputSizes=1
  Data Store Write3 : DataStoreWrite  DataStoreName=LUT_valid  IndexOptions=Index vector (dialog)  Indices=1  OutputSizes=1
  Data Store Write4 : DataStoreWrite  DataStoreName=cal_done  IndexOptions=Index vector (dialog)  Indices=1  OutputSizes=1
  MATLAB Function : MATLAB Function  TreatAsAtomicUnit=on
  wires:
  Data Store Read1/1 -> MATLAB Function/1(k)
  Data Store Read2/1 -> MATLAB Function/2(dphi)
  Data Store Read3/1 -> MATLAB Function/3(phi)
  Data Store Read4/1 -> MATLAB Function/4(varv)
  Data Store Read5/1 -> MATLAB Function/5(cnt)
  Data Store Read6/1 -> MATLAB Function/6(valid)
  Data Store Read7/1 -> MATLAB Function/7(done)
  Constant/1 -> MATLAB Function/8(Nsteady)
  Constant1/1 -> MATLAB Function/9(deadband_rad)
  Constant2/1 -> MATLAB Function/10(var_max)
  Constant3/1 -> MATLAB Function/11(omega_min)
  MATLAB Function/1(phi_n) -> Data Store Write/1
  MATLAB Function/2(varv_n) -> Data Store Write1/1
  MATLAB Function/3(cnt_n) -> Data Store Write2/1
  MATLAB Function/4(valid_n) -> Data Store Write3/1
  MATLAB Function/5(done_n) -> Data Store Write4/1

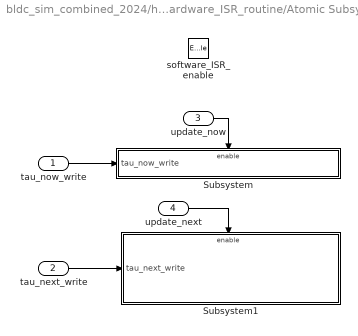
== system bldc_sim_combined_2024/hall_filter/hardware_ISR_routine/Atomic Subsystem ==
  tau_now_write : Inport
  tau_next_write : Inport  Port=2
  update_now : Inport  Port=3
  update_next : Inport  Port=4
  software_ISR_enable : EnablePort
  Subsystem : Subsystem
  Subsystem1 : Subsystem
  wires:
  tau_next_write/1 -> Subsystem1/1(tau_next_write)
  update_now/1 -> Subsystem/Enable
  update_next/1 -> Subsystem1/Enable
  tau_now_write/1 -> Subsystem/1(tau_now_write)

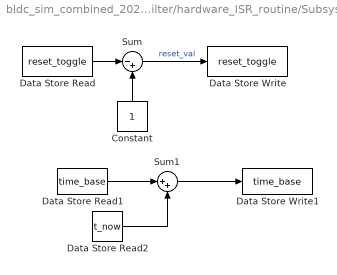
== system bldc_sim_combined_2024/hall_filter/hardware_ISR_routine/Subsystem ==
  Constant : Constant
  Data Store Read : DataStoreRead  DataStoreName=reset_toggle  IndexOptions=Index vector (dialog)  Indices=1  OutputSizes=1
  Data Store Read1 : DataStoreRead  DataStoreName=time_base  IndexOptions=Index vector (dialog)  Indices=1  OutputSizes=1
  Data Store Read2 : DataStoreRead  DataStoreName=t_now  IndexOptions=Index vector (dialog)  Indices=1  OutputSizes=1
  Data Store Write : DataStoreWrite  DataStoreName=reset_toggle  IndexOptions=Index vector (dialog)  Indices=1  OutputSizes=1
  Data Store Write1 : DataStoreWrite  DataStoreName=time_base  IndexOptions=Index vector (dialog)  Indices=1  OutputSizes=1
  Sum : Sum  Inputs=|-+
  Sum1 : Sum  Inputs=|++
  wires:
  Sum/1 -> Data Store Write/1  "reset_val"
  Data Store Read/1 -> Sum/1
  Constant/1 -> Sum/2
  Data Store Read1/1 -> Sum1/1
  Sum1/1 -> Data Store Write1/1
  Data Store Read2/1 -> Sum1/2

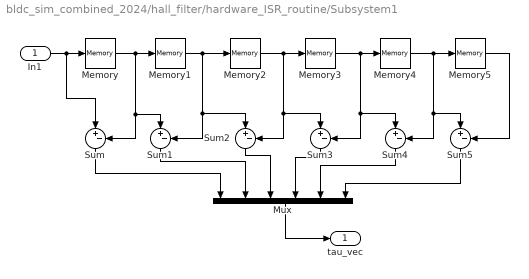
== system bldc_sim_combined_2024/hall_filter/hardware_ISR_routine/Subsystem1 ==
  In1 : Inport
  Memory{,1..5} (6 alike) : Memory  InheritSampleTime=on
  Mux : Mux  Inputs=6
  Sum{,1..5} (6 alike) : Sum  Inputs=|+-
  tau_vec : Outport
  wires:
  Memory1/1 -> Sum1/2, Sum2/1, Memory2/1
  Memory/1 -> Sum1/1, Sum/2, Memory1/1
  Memory2/1 -> Sum3/1, Sum2/2, Memory3/1
  In1/1 -> Sum/1, Memory/1
  Memory3/1 -> Sum4/1, Sum3/2, Memory4/1
  Memory4/1 -> Memory5/1, Sum5/1, Sum4/2
  Mux/1 -> tau_vec/1
  Memory5/1 -> Sum5/2
  Sum/1 -> Mux/1
  Sum1/1 -> Mux/2
  Sum2/1 -> Mux/3
  Sum3/1 -> Mux/4
  Sum4/1 -> Mux/5
  Sum5/1 -> Mux/6

== system bldc_sim_combined_2024/hall_filter/hardware_ISR_routine/Subsystem2 ==
  timer : Inport
  Data Store Write2 : DataStoreWrite  DataStoreName=t_now  IndexOptions=Index vector (dialog)  Indices=1  OutputSizes=1
  wires:
  timer/1 -> Data Store Write2/1

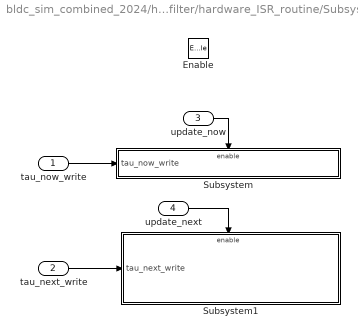
== system bldc_sim_combined_2024/hall_filter/hardware_ISR_routine/Subsystem3 ==
  tau_now_write : Inport
  tau_next_write : Inport  Port=2
  update_now : Inport  Port=3
  update_next : Inport  Port=4
  Enable : EnablePort
  Subsystem : Subsystem
  Subsystem1 : Subsystem
  wires:
  tau_now_write/1 -> Subsystem/1(tau_now_write)
  tau_next_write/1 -> Subsystem1/1(tau_next_write)
  update_now/1 -> Subsystem/Enable
  update_next/1 -> Subsystem1/Enable

== system bldc_sim_combined_2024/hall_filter/software_ISR_routine/Subsystem ==
  Data Store Read : DataStoreRead  DataStoreName=tau_corr_next  IndexOptions=Index vector (dialog)  Indices=1  OutputSizes=1
  Data Store Write : DataStoreWrite  DataStoreName=tau_corr_now  IndexOptions=Index vector (dialog)  Indices=1  OutputSizes=1
  wires:
  Data Store Read/1 -> Data Store Write/1

== system bldc_sim_combined_2024/hall_filter/software_ISR_routine/Subsystem1 ==
  Constant : Constant  Value=-1
  Data Store Write1 : DataStoreWrite  DataStoreName=tau_corr_next  IndexOptions=Index vector (dialog)  Indices=1  OutputSizes=1
  wires:
  Constant/1 -> Data Store Write1/1

== system bldc_sim_combined_2024/hall_filter/software_ISR_routine/Subsystem2 ==
  Constant : Constant
  Data Store Read : DataStoreRead  DataStoreName=state_out  IndexOptions=Index vector (dialog)  Indices=1  OutputSizes=1
  Data Store Write : DataStoreWrite  DataStoreName=state_out  IndexOptions=Index vector (dialog)  Indices=1  OutputSizes=1
  Modulo by Constant : embmathops/Modulo by Constant  Denominator=6  SimulateUsing=Code generation
  Sum : Sum  Inputs=|++
  wires:
  Constant/1 -> Sum/2
  Data Store Read/1 -> Sum/1
  Sum/1 -> Modulo by Constant/1
  Modulo by Constant/1 -> Data Store Write/1

== system bldc_sim_combined_2024/hall_filter/software_ISR_routine/Subsystem3 ==
  Constant : Constant
  Data Store Read : DataStoreRead  DataStoreName=state_out  IndexOptions=Index vector (dialog)  Indices=1  OutputSizes=1
  Sum : Sum  Inputs=|++
  state_out : Outport
  wires:
  Data Store Read/1 -> Sum/1
  Sum/1 -> state_out/1
  Constant/1 -> Sum/2

== system bldc_sim_combined_2024/hall_filter/software_ISR_routine/Subsystem4 ==
  Constant : Constant  Value=0
  Data Store Write : DataStoreWrite  DataStoreName=first_time  IndexOptions=Index vector (dialog)  Indices=1  OutputSizes=1
  wires:
  Constant/1 -> Data Store Write/1

== system bldc_sim_combined_2024/hall_filter/hardware_ISR_routine/Atomic Subsystem/Subsystem ==
  tau_now_write : Inport
  update_now : EnablePort
  Data Store Write : DataStoreWrite  DataStoreName=tau_corr_now  IndexOptions=Index vector (dialog)  Indices=1  OutputSizes=1
  wires:
  tau_now_write/1 -> Data Store Write/1

== system bldc_sim_combined_2024/hall_filter/hardware_ISR_routine/Atomic Subsystem/Subsystem1 ==
  tau_next_write : Inport
  update_next : EnablePort
  Data Store Write1 : DataStoreWrite  DataStoreName=tau_corr_next  IndexOptions=Index vector (dialog)  Indices=1  OutputSizes=1
  wires:
  tau_next_write/1 -> Data Store Write1/1

== system bldc_sim_combined_2024/hall_filter/hardware_ISR_routine/Subsystem3/Subsystem ==
  tau_now_write : Inport
  update_now : EnablePort
  Data Store Write : DataStoreWrite  DataStoreName=tau_corr_now  IndexOptions=Index vector (dialog)  Indices=1  OutputSizes=1
  wires:
  tau_now_write/1 -> Data Store Write/1

== system bldc_sim_combined_2024/hall_filter/hardware_ISR_routine/Subsystem3/Subsystem1 ==
  tau_next_write : Inport
  update_next : EnablePort
  Data Store Write1 : DataStoreWrite  DataStoreName=tau_corr_next  IndexOptions=Index vector (dialog)  Indices=1  OutputSizes=1
  wires:
  tau_next_write/1 -> Data Store Write1/1

== matlab function bldc_sim_combined_2024/hall_filter/MATLAB Function1 ==
  data: interval input; num output
function num = interval_to_num(interval)
DICT = [4,6,2,3,1,5];
if interval == 0
    num = 0;
else
    num = DICT(interval);
end

== matlab function bldc_sim_combined_2024/hall_filter/hardware_ISR_routine/MATLAB Function ==
  data: timer input; tau_now_out output; tau_vec input; tau_now input; tau_next input; tau_next_out output; update_now output; update_next output; tau_corr_out output; tau_LUT_input input; use_LUT input; state_out input
function [tau_now_out, tau_next_out, update_now, update_next, tau_corr_out] = ...
    update_tau_vals_conditional(timer, tau_vec, tau_now, tau_next, ...
                                tau_LUT_input, use_LUT, state_out)

    % 0. Software sector index (0..5)
    persistent sector_idx
    if isempty(sector_idx)
        % Optionally use state_out at startup so you're aligned
        sector_idx = uint8(mod(state_out, 6));  % 0..5
    end

    % 1. Initialize outputs
    tau_now_out  = 0.0;
    tau_next_out = 0.0;
    tau_corr     = 0.0;

    % 2. Compute tau_corr from filter or LUT
    if use_LUT == 1
        % --- LUT MODE: ignore live state_out, use software sector index ---
        tau_corr = tau_LUT_input(sector_idx + 1);   % sector_idx = 0..5
    else
        % --- Quadratic Filter ---
        % tau_corr = (1/3) * ( 4*tau_vec(1) ...
        %                    -    tau_vec(2) ...
        %                    + 2*tau_vec(3) ...
        %                    - 4*tau_vec(4) ...
        %                    + 2*tau_vec(5));

        % --- Six Step Filter ---
        tau_corr = 1/3 * (-tau_vec(1)+tau_vec(3)+tau_vec(4)+tau_vec(5)+tau_vec(6));
    end

    tau_corr_out = tau_corr;

    % 3. Schedule interrupts (unchanged)
    update_now  = false;
    update_next = false;

    if timer <= tau_now
        tau_now_out  = tau_now;          % keep current
        tau_next_out = timer + tau_corr; % schedule next
        update_next  = true;
    else
        tau_now_out  = timer + tau_corr; % schedule now
        tau_next_out = tau_next;         % keep next
        update_now   = true;
    end

    % 4. Advance software sector index once per commutation
    % This function is called once per commutation event, so just walk 0..5.
    if use_LUT == 1
        sector_idx = uint8(mod(double(sector_idx) + 1, 6));
    else
        % In calibration mode you *can* still use state_out if you want to
        % write back into the LUT elsewhere, but here we just leave
        % sector_idx alone or optionally keep it synced:
        % sector_idx = uint8(mod(state_out, 6));
    end
end

== matlab function bldc_sim_combined_2024/hall_filter/calibration_routine/Subsystem2/MATLAB Function ==
  data: k input; phi_n output; dphi input; phi input; varv input; cnt input; valid input; done input; Nsteady input; deadband_rad input; var_max input; omega_min input; varv_n output; cnt_n output; valid_n output; done_n output
function [phi_n,varv_n,cnt_n,valid_n,done_n] = lut_update_one( ...
    k, dphi, phi, varv, cnt, valid, done, ...
    Nsteady, deadband_rad, var_max, omega_min)

% Copy-through defaults
phi_n   = phi;
varv_n  = varv;
cnt_n   = cnt;
valid_n = valid;
done_n  = done;

% Guard: out-of-range index or already done
if done || k < 1 || k > 6
    return;
end

% ---- Welford mean/variance update for entry k ----
n  = double(cnt(k));
mu = double(phi(k));
M2 = double(varv(k)) * max(n - 1, 0);

n  = n + 1;
if n == 1
    mu = double(dphi);
    M2 = 0.0;
else
    delta = double(dphi) - mu;
    mu    = mu + delta / n;
    M2    = M2 + delta * (double(dphi) - mu);
end

cnt_n(k)  = uint8(min(n, 255));
phi_n(k)  = single(mu);
if n > 1
    varv_n(k) = single(M2 / (n - 1));
else
    varv_n(k) = single(0);
end

% ---- Validity for this state ----
close_ok = (abs(double(dphi) - mu) <= double(deadband_rad));
var_ok   = (double(varv_n(k))      <= double(var_max));
count_ok = (n >= double(Nsteady));
if close_ok && var_ok && count_ok
    valid_n(k) = true;
end

% ---- Global done ----
allv = true;
for i = 1:6
    allv = allv && valid_n(i);
end
if allv
    done_n = true;
end

== matlab function bldc_sim_combined_2024/hall_filter/hardware_ISR_routine/MATLAB Function1 ==
  data: tau_LUT_input input; tau_corr_LUT_test output
function tau_corr_LUT_test = tau_corr_LUT_test_fn(tau_LUT_input)
%#codegen
% tau_LUT_input : 6x1 or 1x6 vector of tau values for sectors 0..5
% use_LUT       : scalar flag (0/1), lets you freeze counter in filter mode

    % Software sector index (0..5), independent of Hall state
    persistent sector_idx
    if isempty(sector_idx)
        sector_idx = uint8(0);  % internal counter 0..5
    end

    % --- sector phase offset in "steps" (−1 step == +5 mod 6) ---
    % Adjust this if you find it leads instead of lags.
    offset = int8(-1);    % one-sector *earlier* than the counter
    % offset = +1 would be one-sector later, etc.

    % Default output
    tau_corr_LUT_test = 0.0;

    % Compute current LUT index with phase offset
    k = int8(sector_idx) + offset;       % may be negative
    k = mod(double(k), 6);               % wrap into 0..5
    idx = uint8(k) + 1;                  % 1-based for MATLAB

    % Use LUT entry
    tau_corr_LUT_test = tau_LUT_input(idx);

    % Only advance the counter when LUT mode is active

        sector_idx = uint8(mod(double(sector_idx) + 1, 6));
    
end

== matlab function bldc_sim_combined_2024/qd-frame to stator ==
  data: fa output; fb output; fc output; fq input; fd input; theta input
function [fa,fb,fc] = K_mat_inv_sim(fq,fd,theta)
[fa,fb,fc] = K_mat_inv(fq,fd,theta);

== matlab function bldc_sim_combined_2024/stator to qd-frame ==
  data: fa input; fq output; fb input; fc input; theta input; fd output
function [fq,fd] = K_mat_sim(fa,fb,fc,theta)
[fq,fd] = K_mat(fa,fb,fc,theta);

== matlab function bldc_sim_combined_2024/controller_1 ==
  data: HALL_STATE input; T_vec output
function T_vec = controller_6step_120_sim(HALL_STATE)
T_vec = controller_6step_120(HALL_STATE);
end

== matlab function bldc_sim_combined_2024/hall sensors ==
  data: hall_errors input; theta_r input; H1 output; H2 output; H3 output
function [H1,H2,H3] = hall_sensor_sim(hall_errors, theta_r)
[H1,H2,H3] = hall_sensor(theta_r, hall_errors);
end
